simulink model "RPI1DesktopValidation"  (R2026a)
settings: Solver=FixedStepDiscrete  StopTime=60  FixedStep=rccar.SampleTime
InitFcn:
  | rccarRoot=fileparts(fileparts(fileparts(get_param(bdroot,'FileName')))); addpath(genpath(rccarRoot)); setupRCCarProject; clear rccarRoot;
undefined symbols (not defined in the file): f, rccar
libraries: instrumentlib x1
settings Model: Creator=taegon  LastModifiedBy=taegon

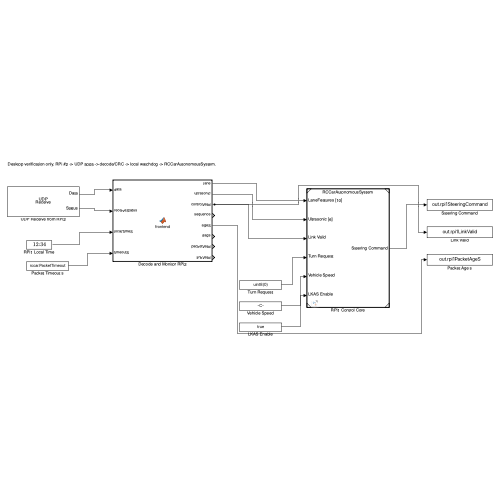
[thumbnail: Simulink's stored preview of the top-level diagram]
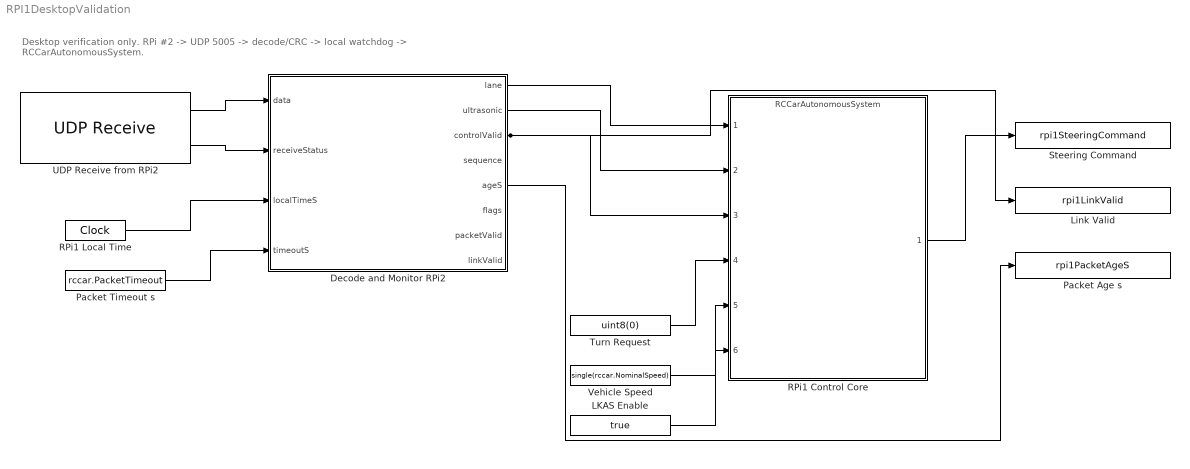
== system RPI1DesktopValidation ==
  note: Desktop verification only. RPi #2 -> UDP 5005 -> decode/CRC -> local watchdog -> RCCarAutonomousSystem.
  Decode and Monitor RPi2 : MATLAB Function  TreatAsAtomicUnit=on
  LKAS Enable : Constant  Value=true  OutDataTypeStr=boolean
  Link Valid : ToWorkspace  VariableName=rpi1LinkValid  SaveFormat=Timeseries  SampleTime=-1
  Packet Age s : ToWorkspace  VariableName=rpi1PacketAgeS  SaveFormat=Timeseries  SampleTime=-1
  Packet Timeout s : Constant  Value=rccar.PacketTimeout  OutDataTypeStr=double
  RPi1 Control Core : ModelReference  ModelNameDialog=RCCarAutonomousSystem  SimulationMode=Normal  ModelReferenceVersion=1.3
  RPi1 Local Time : DigitalClock  SampleTime=rccar.SampleTime
  Steering Command : ToWorkspace  VariableName=rpi1SteeringCommand  SaveFormat=Timeseries  SampleTime=-1
  Turn Request : Constant  Value=uint8(0)  OutDataTypeStr=uint8
  UDP Receive from RPi2 : instrumentlib/UDP Receive  LocalAddress=0.0.0.0  LocalPort=5005  EnablePortSharing=off  Host=192.168.202.104  Port=5006  GetLatestData=on  DataSize=[80 1]  DataType=uint8  ASCIIFormatting=%f,  Terminator=LF  CustomTerminator=10  ByteOrder=little-endian  EnableBlockingMode=off  Timeout=10  SampleTime=rccar.SampleTime  SimulateUsing=Interpreted execution
  Vehicle Speed : Constant  Value=single(rccar.NominalSpeed)  OutDataTypeStr=single
  wires:
  UDP Receive from RPi2/1 -> Decode and Monitor RPi2/1(data)
  UDP Receive from RPi2/2 -> Decode and Monitor RPi2/2(receiveStatus)
  RPi1 Local Time/1 -> Decode and Monitor RPi2/3(localTimeS)
  Packet Timeout s/1 -> Decode and Monitor RPi2/4(timeoutS)
  Decode and Monitor RPi2/1(lane) -> RPi1 Control Core/1
  Decode and Monitor RPi2/2(ultrasonic) -> RPi1 Control Core/2
  Decode and Monitor RPi2/3(controlValid) -> RPi1 Control Core/3, Link Valid/1
  Turn Request/1 -> RPi1 Control Core/4
  Vehicle Speed/1 -> RPi1 Control Core/5
  LKAS Enable/1 -> RPi1 Control Core/6
  RPi1 Control Core/1 -> Steering Command/1
  Decode and Monitor RPi2/5(ageS) -> Packet Age s/1

== matlab function RPI1DesktopValidation/Decode and Monitor RPi2 ==
  data: data input uint8 size=[80 1]; lane output single size=[10 1]; receiveStatus input boolean size=1; localTimeS input double size=1; timeoutS input double size=1; ultrasonic output single size=[6 1]; controlValid output boolean size=1; sequence output uint32 size=1; ageS output double size=1; flags output uint8 size=1; packetValid output boolean size=1; linkValid output boolean size=1
function [lane, ultrasonic, controlValid, sequence, ageS, flags, packetValid, linkValid] = frontend(data, receiveStatus, localTimeS, timeoutS)
%#codegen
persistent heldLane heldSide heldFlags heldSequence
if isempty(heldLane)
 heldLane=zeros(10,1,'single'); heldSide=single([NaN;NaN]);
 heldFlags=uint8(0); heldSequence=uint32(0);
end
[newLane,newSide,newFlags,newSequence,~,~,packetValid]=rpi2DecodePacket(data,receiveStatus);
if packetValid
 heldLane=newLane; heldSide=newSide; heldFlags=newFlags; heldSequence=newSequence;
end
[linkValid,ageS,~]=rpi2LinkMonitor(localTimeS,packetValid,newSequence,timeoutS,false);
cameraValid=bitand(heldFlags,uint8(1))~=0; laneValid=bitand(heldFlags,uint8(2))~=0;
controlValid=linkValid && cameraValid && laneValid;
lane=heldLane; ultrasonic=single([NaN;NaN;heldSide(1);heldSide(2);NaN;NaN]);
sequence=heldSequence; flags=heldFlags;
end
